simulink model "RootLocus_controller"  (R2021b)
settings: Solver=ode45  StartTime=0.0  StopTime=1  RelTol=1e-3
values from neighbouring files (symbols this model uses):
  Gd_RL = K*PI*PD    [Project.m]
  Gs = G1 * G2    [Project.m]
  Ts = 0.02    [Project.m]
settings Model: Creator=Amir  LastModifiedBy=Amir

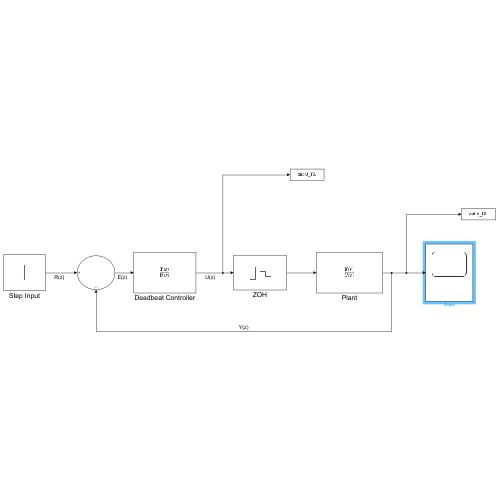
[thumbnail: Simulink's stored preview of the top-level diagram]
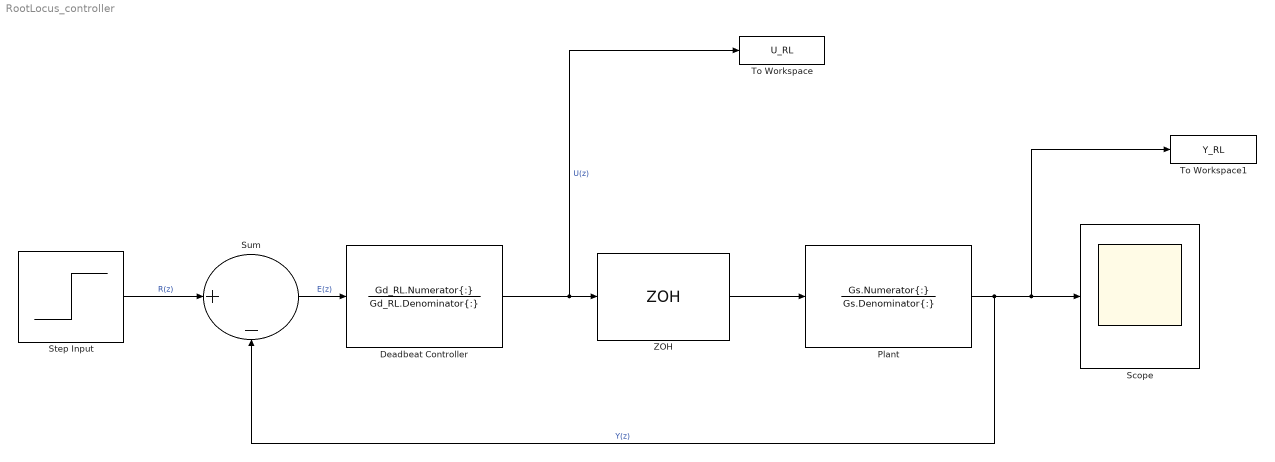
== system RootLocus_controller ==
  Deadbeat Controller : DiscreteTransferFcn  Numerator=Gd_RL.Numerator{:}  Denominator=Gd_RL.Denominator{:}  SampleTime=Ts
  Plant : TransferFcn  Numerator=Gs.Numerator{:}  Denominator=Gs.Denominator{:}
  Scope : Scope
  Step Input : Step  Time=0  After=0.01  SampleTime=0
  Sum : Sum  Inputs=|+-
  To Workspace : ToWorkspace  VariableName=U_RL  SaveFormat=Timeseries  SampleTime=-1
  To Workspace1 : ToWorkspace  VariableName=Y_RL  SaveFormat=Timeseries  SampleTime=-1
  ZOH : ZeroOrderHold  SampleTime=Ts
  wires:
  Deadbeat Controller/1 -> To Workspace/1, ZOH/1  "U(z)"
  ZOH/1 -> Plant/1
  Plant/1 -> Sum/2, To Workspace1/1, Scope/1  "Y(z)"
  Step Input/1 -> Sum/1  "R(z)"
  Sum/1 -> Deadbeat Controller/1  "E(z)"
